simulink model "Urban_Air_Mobility_v3"  (R2021a)
settings: Solver=ode4  StartTime=0.0  StopTime=50  FixedStep=0.01  RelTol=1e-3
model workspace (MAT data in the model file):
  op_trim2 : handle (value not decoded)
undefined symbols (not defined in the file or in its folder): BackProp, Earth, ForwProp, geo, initialise, mass, simsetup, WGS84
libraries: dspindex x6, aerolibactuator x4, sharedutil x3, simulink x3, aerolibasang x2, aerolibtransform2 x2, aerolibutil x2, shared6dof x1, aerolibatmos2 x1, sharedtransform x1, aerolibconvert2 x1
(part 1 of 3)
settings Model: Creator=c109799  LastModifiedBy=gonza
settings SolverCC: AlgebraicLoopSolver=TrustRegion
settings DataIOCC: ExternalInput=getinputstruct(op_trim1)  InitialState=getstatestruct(op_trim1)  LoadExternalInput=on  LoadInitialState=on
settings DebuggingCC: SFMachineParentedDataDiag=warning  ArithmeticOperatorsInVariantConditions=warning
settings SFSimCC: CustomCodeUndefinedFunction=UseInterfaceOnly

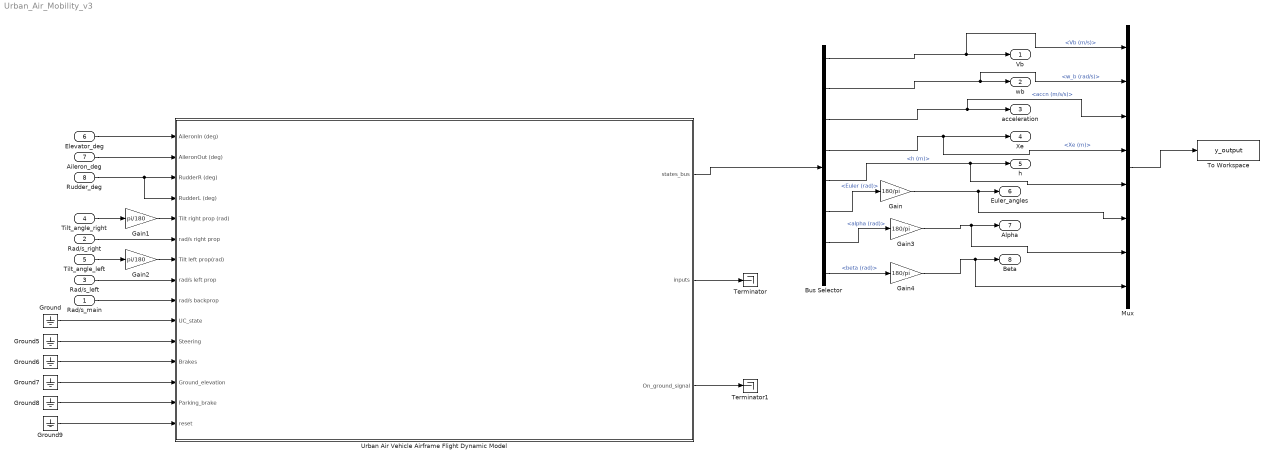
== system Urban_Air_Mobility_v3 ==
  Rad/s_main : Inport
  Rad/s_right : Inport  Port=2
  Rad/s_left : Inport  Port=3
  Tilt_angle_right : Inport  Port=4
  Tilt_angle_left : Inport  Port=5
  Elevator_deg : Inport  Port=6
  Aileron_deg : Inport  Port=7
  Rudder_deg : Inport  Port=8
  Bus Selector : BusSelector  OutputSignals=Vb (m/s),w_b (rad/s),accn (m/s/s),Xe (m),h (m),Euler (rad),alpha (rad),beta (rad)
  Gain : Gain  Gain=180/pi
  Gain1 : Gain  Gain=pi/180
  Gain2 : Gain  Gain=pi/180
  Gain3 : Gain  Gain=180/pi
  Gain4 : Gain  Gain=180/pi
  Ground{,5..9} (6 alike) : Ground
  Mux : Mux  Inputs=8
  Terminator : Terminator
  Terminator1 : Terminator
  To Workspace : ToWorkspace  VariableName=y_output  SampleTime=-1
  Urban Air Vehicle Airframe Flight Dynamic Model : Subsystem
  Vb : Outport  VectorParamsAs1DForOutWhenUnconnected=off
  wb : Outport  Port=2  VectorParamsAs1DForOutWhenUnconnected=off
  acceleration : Outport  Port=3  VectorParamsAs1DForOutWhenUnconnected=off
  Xe : Outport  Port=4  VectorParamsAs1DForOutWhenUnconnected=off
  h : Outport  Port=5  VectorParamsAs1DForOutWhenUnconnected=off
  Euler_angles : Outport  Port=6  VectorParamsAs1DForOutWhenUnconnected=off
  Alpha : Outport  Port=7  VectorParamsAs1DForOutWhenUnconnected=off
  Beta : Outport  Port=8  VectorParamsAs1DForOutWhenUnconnected=off
  wires:
  Ground/1 -> Urban Air Vehicle Airframe Flight Dynamic Model/10(UC_state)
  Ground5/1 -> Urban Air Vehicle Airframe Flight Dynamic Model/11(Steering)
  Ground6/1 -> Urban Air Vehicle Airframe Flight Dynamic Model/12(Brakes)
  Ground7/1 -> Urban Air Vehicle Airframe Flight Dynamic Model/13(Ground_elevation)
  Ground8/1 -> Urban Air Vehicle Airframe Flight Dynamic Model/14(Parking_brake)
  Ground9/1 -> Urban Air Vehicle Airframe Flight Dynamic Model/15("reset ")
  Urban Air Vehicle Airframe Flight Dynamic Model/1(states_bus) -> Bus Selector/1
  Urban Air Vehicle Airframe Flight Dynamic Model/2(inputs) -> Terminator/1
  Urban Air Vehicle Airframe Flight Dynamic Model/3(On_ground_signal) -> Terminator1/1
  Bus Selector/2 -> Mux/2, wb/1  "<w_b (rad/s)>"
  Bus Selector/5 -> Mux/5, h/1  "<h (m)>"
  Bus Selector/6 -> Gain/1  "<Euler (rad)>"
  Gain/1 -> Mux/6, Euler_angles/1
  Rudder_deg/1 -> Urban Air Vehicle Airframe Flight Dynamic Model/4("RudderL (deg) "), Urban Air Vehicle Airframe Flight Dynamic Model/3(RudderR (deg))
  Rad/s_main/1 -> Urban Air Vehicle Airframe Flight Dynamic Model/9(rad/s backprop)
  Rad/s_right/1 -> Urban Air Vehicle Airframe Flight Dynamic Model/6(rad/s right prop)
  Bus Selector/1 -> Mux/1, Vb/1  "<Vb (m/s)>"
  Bus Selector/3 -> Mux/3, acceleration/1  "<accn (m/s/s)>"
  Bus Selector/4 -> Mux/4, Xe/1  "<Xe (m)>"
  Aileron_deg/1 -> Urban Air Vehicle Airframe Flight Dynamic Model/2(AileronOut (deg))
  Elevator_deg/1 -> Urban Air Vehicle Airframe Flight Dynamic Model/1(AileronIn (deg))
  Gain1/1 -> Urban Air Vehicle Airframe Flight Dynamic Model/5(Tilt right prop (rad))
  Tilt_angle_right/1 -> Gain1/1
  Gain2/1 -> Urban Air Vehicle Airframe Flight Dynamic Model/7(Tilt left prop(rad))
  Tilt_angle_left/1 -> Gain2/1
  Bus Selector/7 -> Gain3/1  "<alpha (rad)>"
  Gain3/1 -> Mux/7, Alpha/1
  Bus Selector/8 -> Gain4/1  "<beta (rad)>"
  Gain4/1 -> Mux/8, Beta/1
  Mux/1 -> To Workspace/1
  Rad/s_left/1 -> Urban Air Vehicle Airframe Flight Dynamic Model/8(rad/s left prop)

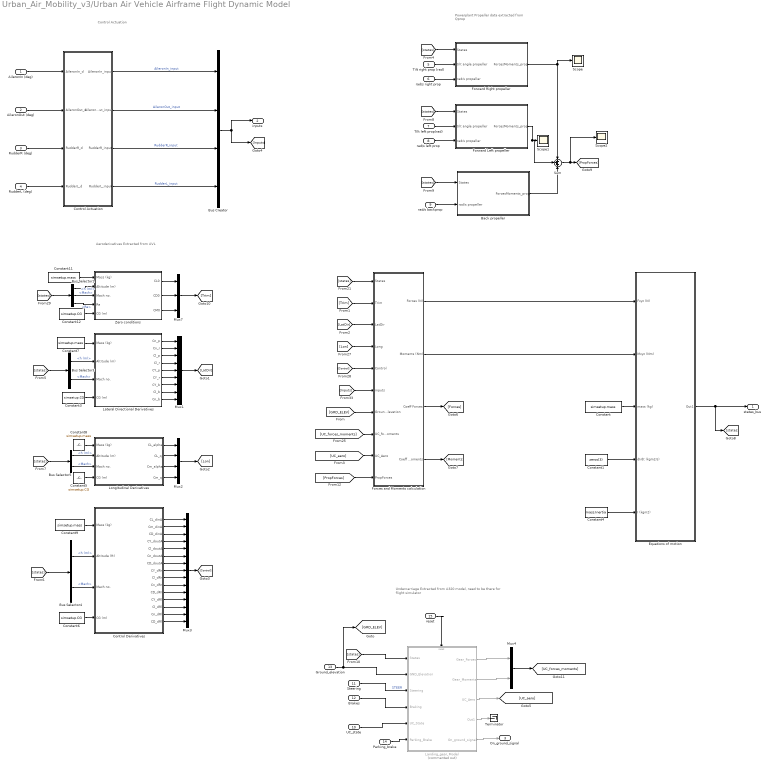
== system Urban_Air_Mobility_v3/Urban Air Vehicle Airframe Flight Dynamic Model ==
  note: Undercarriage
      | Extracted from A320 model, need to be there for flight simulator
  note: Control Actuation
  note: Aeroderivatives
      | Extracted from AVL
  note: Powerplant
      | Propeller data extracted from Qprop
  AileronIn (deg) : Inport
  AileronOut (deg) : Inport  Port=2
  RudderR (deg) : Inport  Port=3
  "RudderL (deg) " : Inport  Port=4
  Tilt right prop (rad) : Inport  Port=5
  rad/s right prop : Inport  Port=6
  Tilt left prop(rad) : Inport  Port=7
  rad/s left prop : Inport  Port=8
  rad/s backprop : Inport  Port=9
  UC_state : Inport  Port=10
  Steering : Inport  Port=11
  Brakes : Inport  Port=12
  Ground_elevation : Inport  Port=13
  Parking_brake : Inport  Port=14
  "reset " : Inport  Port=15
  Back propeller : Subsystem
  Bus Creator : BusCreator  Inputs=4
  Bus Selector1 : BusSelector  OutputSignals=h (m),Mach,Re
  Bus Selector3 : BusSelector  OutputSignals=h (m),Mach
  Bus Selector4 : BusSelector  OutputSignals=h (m),Mach
  Bus Selector5 : BusSelector  OutputSignals=h (m),Mach
  Constant{,7..9,11} (5 alike) : Constant  Value=simsetup.mass
  Constant1 : Constant  Value=zeros(3)
  Constant{3,5..6,12} (4 alike) : Constant  Value=simsetup.CG
  Constant4 : Constant  Value=mass.Inertia
  Control Actuation : Subsystem
  Control Derivatives : Subsystem
  Equations of motion : Subsystem
  Forces and Moments calculation : Subsystem
  Forward Left propeller : Subsystem
  Forward Right propeller : Subsystem
  Landing_gear_Model : Subsystem  Commented=on
  Lateral Directional Derivatives : Subsystem
  Longitudinal Derivatives : Subsystem
  Mux1 : Mux  Inputs=9
  Mux2 : Mux
  Mux3 : Mux  Inputs=15
  Mux4 : Mux  Inputs=2
  Mux7 : Mux  Inputs=3
  Scope : Scope
  Scope1 : Scope
  Scope2 : Scope
  Sum : Sum  Inputs=+++
  Terminator : Terminator
  Zero conditions : Subsystem
  states_bus : Outport  VectorParamsAs1DForOutWhenUnconnected=off
  inputs : Outport  Port=2  VectorParamsAs1DForOutWhenUnconnected=off
  On_ground_signal : Outport  Port=3  VectorParamsAs1DForOutWhenUnconnected=off
  wires:
  RudderR (deg)/1 -> Control Actuation/3(RudderR_d)
  Bus Creator/1 -> inputs/1, [Inputs]
  Lateral Directional Derivatives/5(CY_p) -> Mux1/5
  Lateral Directional Derivatives/6(CY_r) -> Mux1/6
  [states] -> Bus Selector4/1
  Bus Selector5/1 -> Longitudinal Derivatives/2(Altitude (m))  "<h (m)>"
  Mux2/1 -> [Lon]
  Bus Selector3/2 -> Lateral Directional Derivatives/3(Mach no.)  "<Mach>"
  Longitudinal Derivatives/4(Cm_q) -> Mux2/4
  Lateral Directional Derivatives/8(Cl_b) -> Mux1/8
  Bus Selector4/2 -> Control Derivatives/3(Mach no.)  "<Mach>"
  Lateral Directional Derivatives/4(Cl_r) -> Mux1/4
  Constant7/1 -> Lateral Directional Derivatives/1(Mass (kg))
  Lateral Directional Derivatives/3(Cl_p) -> Mux1/3
  Constant8/1 -> Longitudinal Derivatives/1(Mass (kg))
  Bus Selector3/1 -> Lateral Directional Derivatives/2(Altitude (m))  "<h (m)>"
  Bus Selector4/1 -> Control Derivatives/2(Altitude (ft))  "<h (m)>"
  [states] -> Bus Selector5/1
  Constant9/1 -> Control Derivatives/1(Mass (kg))
  Mux1/1 -> [LatDir]
  Longitudinal Derivatives/2(CL_q) -> Mux2/2
  Longitudinal Derivatives/3(Cm_alpha) -> Mux2/3
  Constant5/1 -> Longitudinal Derivatives/4(CG (m))
  Mux3/1 -> [Control]
  Lateral Directional Derivatives/1(Cn_p) -> Mux1/1
  Longitudinal Derivatives/1(CL_alpha) -> Mux2/1
  Lateral Directional Derivatives/7(CY_b) -> Mux1/7
  [states] -> Bus Selector3/1
  Constant6/1 -> Control Derivatives/4(CG (m))
  Constant3/1 -> Lateral Directional Derivatives/4(CG (m))
  Lateral Directional Derivatives/2(Cn_r) -> Mux1/2
  Bus Selector5/2 -> Longitudinal Derivatives/3(Mach no.)  "<Mach>"
  Equations of motion/1(Out1) -> [states], states_bus/1
  AileronIn (deg)/1 -> Control Actuation/1("AileronIn_d ")
  [UC_forces_moments] -> Forces and Moments calculation/8(UC_forces_moments)
  [Control] -> Forces and Moments calculation/5(Control)
  Forces and Moments calculation/4(Coeff Moments) -> [Moments]
  [Inputs] -> Forces and Moments calculation/6(inputs)
  [LatDir] -> Forces and Moments calculation/3(LatDir)
  Forces and Moments calculation/3(Coeff Forces) -> [Forces]
  [Lon] -> Forces and Moments calculation/4(Long)
  [Trim] -> Forces and Moments calculation/2(Trim)
  [states] -> Forces and Moments calculation/1(States)
  [states] -> Landing_gear_Model/1(States)
  Steering/1 -> Landing_gear_Model/3(Steering)  "STEER"
  Brakes/1 -> Landing_gear_Model/4(Braking)
  Ground_elevation/1 -> [GRD_ELEV], Landing_gear_Model/2(GND_Elevation)
  UC_state/1 -> Landing_gear_Model/5(UC_State)
  Mux4/1 -> [UC_forces_moments]
  Forces and Moments calculation/1(Forces (N)) -> Equations of motion/1(Fxyz (N))
  Forces and Moments calculation/2(Moments (Nm)) -> Equations of motion/2(Mxyz (Nm))
  Landing_gear_Model/3(UC_Aero) -> [UC_aero]
  Control Actuation/3(RudderR_input) -> Bus Creator/3  "RudderR_input"
  Landing_gear_Model/2(Gear_Moments) -> Mux4/2
  Landing_gear_Model/1(Gear_Forces) -> Mux4/1
  [GRD_ELEV] -> Forces and Moments calculation/7(Ground_Elevation)
  Parking_brake/1 -> Landing_gear_Model/6(Parking_Brake)
  Landing_gear_Model/5(On_ground_signal) -> On_ground_signal/1
  "reset "/1 -> Landing_gear_Model/Reset
  Landing_gear_Model/4(Out1) -> Terminator/1
  Constant/1 -> Equations of motion/3(mass (kg))
  Constant1/1 -> Equations of motion/4(dI/dt (kgm2/s))
  Constant4/1 -> Equations of motion/5(I (kgm2))
  [UC_aero] -> Forces and Moments calculation/9(UC_Aero)
  Lateral Directional Derivatives/9(Cn_b) -> Mux1/9
  Control Derivatives/1(CL_dinA) -> Mux3/1
  Control Derivatives/2(Cm_dinA) -> Mux3/2
  Control Derivatives/3(CD_dinA) -> Mux3/3
  AileronOut (deg)/1 -> Control Actuation/2(AileronOut_d)
  "RudderL (deg) "/1 -> Control Actuation/4("RudderL_d ")
  Control Actuation/1(AileronIn_input) -> Bus Creator/1  "AileronIn_input"
  Control Actuation/2(AileronOut_input) -> Bus Creator/2  "AileronOut_input"
  Control Actuation/4(RudderL_input) -> Bus Creator/4  "RudderL_input"
  Control Derivatives/4(CY_doutA) -> Mux3/4
  Control Derivatives/5(Cl_doutA) -> Mux3/5
  Control Derivatives/6(Cn_doutA) -> Mux3/6
  Control Derivatives/14(Cn_dRl) -> Mux3/14
  Control Derivatives/15(CD_dRl) -> Mux3/15
  Control Derivatives/13(Cl_dRl) -> Mux3/13
  Control Derivatives/12(CY_dRl) -> Mux3/12
  Control Derivatives/11(CD_dRr) -> Mux3/11
  Control Derivatives/10(Cn_dRr) -> Mux3/10
  Control Derivatives/9(Cl_dRr) -> Mux3/9
  Control Derivatives/8(CY_dRr) -> Mux3/8
  Control Derivatives/7(CD_doutA) -> Mux3/7
  [PropForces] -> Forces and Moments calculation/10(PropForces)
  Forward Right propeller/1(ForcesMoments_prop) -> Scope/1, Sum/1
  Forward Left propeller/1(ForcesMoments_prop) -> Sum/2, Scope1/1
  Sum/1 -> Scope2/1, [PropForces]
  [states] -> Forward Right propeller/1(States)
  Tilt left prop(rad)/1 -> Forward Left propeller/2(tilt angle propeller)
  rad/s right prop/1 -> Forward Right propeller/3(rad/s propeller)
  Tilt right prop (rad)/1 -> Forward Right propeller/2(tilt angle propeller)
  rad/s backprop/1 -> Back propeller/2(rad/s propeller)
  [states] -> Back propeller/1(States)
  rad/s left prop/1 -> Forward Left propeller/3(rad/s propeller)
  [states] -> Forward Left propeller/1(States)
  Back propeller/1(ForcesMoments_prop) -> Sum/3
  Zero conditions/3(CM0) -> Mux7/3
  Zero conditions/1(CL0) -> Mux7/1
  Bus Selector1/1 -> Zero conditions/2(Altitude (m))  "<h (m)>"
  Constant12/1 -> Zero conditions/5(CG (m))
  Zero conditions/2(CD0) -> Mux7/2
  [states] -> Bus Selector1/1
  Bus Selector1/2 -> Zero conditions/3(Mach no.)  "<Mach>"
  Mux7/1 -> [Trim]
  Bus Selector1/3 -> Zero conditions/4(Re)  "<Re>"
  Constant11/1 -> Zero conditions/1(Mass (kg))

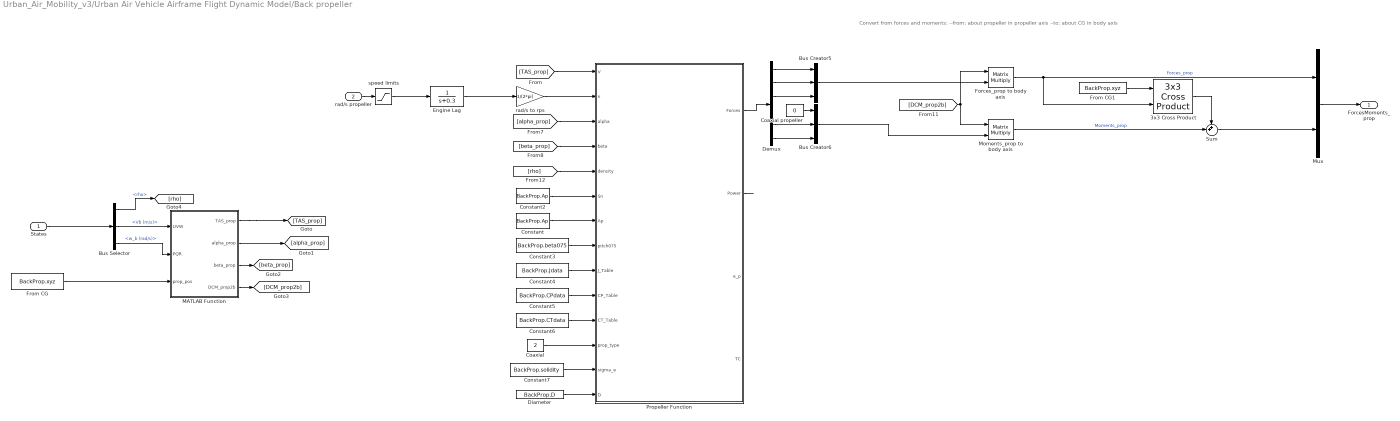
== system Urban_Air_Mobility_v3/Urban Air Vehicle Airframe Flight Dynamic Model/Back propeller ==
  note: Convert from forces and moments: --from: about propeller in propeller axis --to: about CG in body axis
  States : Inport
  rad/s propeller : Inport  Port=2
  3x3 Cross Product : sharedutil/3x3 Cross Product  aMode=aMode
      settings: SourceProductBaseCode=AE,PW,DR,MT,UV,VE
  Bus Creator5 : BusCreator  Inputs=3
  Bus Creator6 : BusCreator  Inputs=3
  Bus Selector : BusSelector  OutputSignals=rho,Vb (m/s),w_b (rad/s)
  "Coaxial " : Constant  Value=2
  Coaxial propeller : Constant  Value=0
  Constant : Constant  Value=BackProp.Ap
  Constant2 : Constant  Value=BackProp.Ap
  Constant3 : Constant  Value=BackProp.beta075
  Constant4 : Constant  Value=BackProp.Jdata
  Constant5 : Constant  Value=BackProp.CPdata
  Constant6 : Constant  Value=BackProp.CTdata
  Constant7 : Constant  Value=BackProp.solidity
  Demux : Demux  Outputs=6
  Diameter : Constant  Value=BackProp.D
  Engine Lag : TransferFcn  Denominator=[1 0.3]  ContinuousStateAttributes='EngineLag'
  Forces_prop to body axis : Product  Multiplication=Matrix(*)
  From CG : Constant  Value=BackProp.xyz
  From CG1 : Constant  Value=BackProp.xyz
  MATLAB Function : MATLAB Function  TreatAsAtomicUnit=on
  Moments_prop to body axis : Product  Multiplication=Matrix(*)
  Mux : Mux  Inputs=2
  Propeller Function : MATLAB Function  TreatAsAtomicUnit=on
  Sum : Sum  Inputs=++|
  rad/s to rps : Gain  Gain=1/(2*pi)
  speed limits : Saturate  UpperLimit=2000  LowerLimit=-1500
  ForcesMoments_prop : Outport
  wires:
  [rho] -> Propeller Function/5(density)
  MATLAB Function/2(alpha_prop) -> [alpha_prop]
  MATLAB Function/3(beta_prop) -> [beta_prop]
  MATLAB Function/1(TAS_prop) -> [TAS_prop]
  MATLAB Function/4(DCM_prop2b) -> [DCM_prop2b]
  [TAS_prop] -> Propeller Function/1(V)
  From CG/1 -> MATLAB Function/3(prop_pos)
  [alpha_prop] -> Propeller Function/3(alpha)
  rad/s propeller/1 -> speed limits/1
  States/1 -> Bus Selector/1
  Bus Selector/2 -> MATLAB Function/1(UVW)  "<Vb (m/s)>"
  Bus Selector/3 -> MATLAB Function/2(PQR)  "<w_b (rad/s)>"
  Bus Selector/1 -> [rho]  "<rho>"
  Mux/1 -> ForcesMoments_prop/1
  3x3 Cross Product/1 -> Sum/1
  Moments_prop to body axis/1 -> Sum/2  "Moments_prop"
  Forces_prop to body axis/1 -> 3x3 Cross Product/2, Mux/1  "Forces_prop"
  [DCM_prop2b] -> Forces_prop to body axis/1, Moments_prop to body axis/1
  From CG1/1 -> 3x3 Cross Product/1
  Bus Creator6/1 -> Moments_prop to body axis/2
  Sum/1 -> Mux/2
  [beta_prop] -> Propeller Function/4(beta)
  Constant/1 -> Propeller Function/7(Ap)
  Constant2/1 -> Propeller Function/6(Sn)
  Constant3/1 -> Propeller Function/8(pitch075)
  Constant4/1 -> Propeller Function/9(J_Table)
  Constant5/1 -> Propeller Function/10(CP_Table)
  Constant6/1 -> Propeller Function/11(CT_Table)
  Constant7/1 -> Propeller Function/13(sigma_e)
  "Coaxial "/1 -> Propeller Function/12(prop_type)
  Propeller Function/1(Forces) -> Demux/1
  Demux/1 -> Bus Creator5/1
  Demux/6 -> Bus Creator6/3
  Demux/2 -> Bus Creator5/2
  Demux/3 -> Bus Creator5/3
  Demux/5 -> Bus Creator6/2
  Propeller Function/2(Power) -> ?
  speed limits/1 -> Engine Lag/1
  Engine Lag/1 -> rad/s to rps/1
  Diameter/1 -> Propeller Function/14(D)
  rad/s to rps/1 -> Propeller Function/2(n)
  Coaxial propeller/1 -> Bus Creator6/1
  Bus Creator5/1 -> Forces_prop to body axis/2

== system Urban_Air_Mobility_v3/Urban Air Vehicle Airframe Flight Dynamic Model/Control Actuation ==
  "AileronIn_d " : Inport
  AileronOut_d : Inport  Port=2
  RudderR_d : Inport  Port=3
  "RudderL_d " : Inport  Port=4
  Aileron Actuator Transfer Function1 : aerolibactuator/Nonlinear Second-Order Actuator  wn_fin=45  z_fin=0.8  fin_max=25*pi/180  fin_min=-25*pi/180  fin_maxrate=100*pi/180  fin_act_0=0  fin_act_vel=0
      settings: SourceProductBaseCode=AE
  Aileron Actuator Transfer Function2 : aerolibactuator/Nonlinear Second-Order Actuator  wn_fin=45  z_fin=0.8  fin_max=25*pi/180  fin_min=-25*pi/180  fin_maxrate=100*pi/180  fin_act_0=0  fin_act_vel=0
      settings: SourceProductBaseCode=AE
  Rudder  Actuator Transfer Function1 : aerolibactuator/Nonlinear Second-Order Actuator  wn_fin=45  z_fin=0.8  fin_max=25*pi/180  fin_min=-25*pi/180  fin_maxrate=100*pi/180  fin_act_0=0  fin_act_vel=0
      settings: SourceProductBaseCode=AE
  Rudder  Actuator Transfer Function2 : aerolibactuator/Nonlinear Second-Order Actuator  wn_fin=45  z_fin=0.8  fin_max=25*pi/180  fin_min=-25*pi/180  fin_maxrate=100*pi/180  fin_act_0=0  fin_act_vel=0
      settings: SourceProductBaseCode=AE
  AileronIn_input : Outport  VectorParamsAs1DForOutWhenUnconnected=off
  AileronOut_input : Outport  Port=2  VectorParamsAs1DForOutWhenUnconnected=off
  RudderR_input : Outport  Port=3  VectorParamsAs1DForOutWhenUnconnected=off
  RudderL_input : Outport  Port=4  VectorParamsAs1DForOutWhenUnconnected=off
  wires:
  "AileronIn_d "/1 -> Aileron Actuator Transfer Function1/1
  RudderR_d/1 -> Rudder  Actuator Transfer Function1/1
  Aileron Actuator Transfer Function1/1 -> AileronIn_input/1  "Elevator_input"
  Rudder  Actuator Transfer Function1/1 -> RudderR_input/1
  AileronOut_d/1 -> Aileron Actuator Transfer Function2/1
  Aileron Actuator Transfer Function2/1 -> AileronOut_input/1  "Aileron_input"
  Rudder  Actuator Transfer Function2/1 -> RudderL_input/1
  "RudderL_d "/1 -> Rudder  Actuator Transfer Function2/1

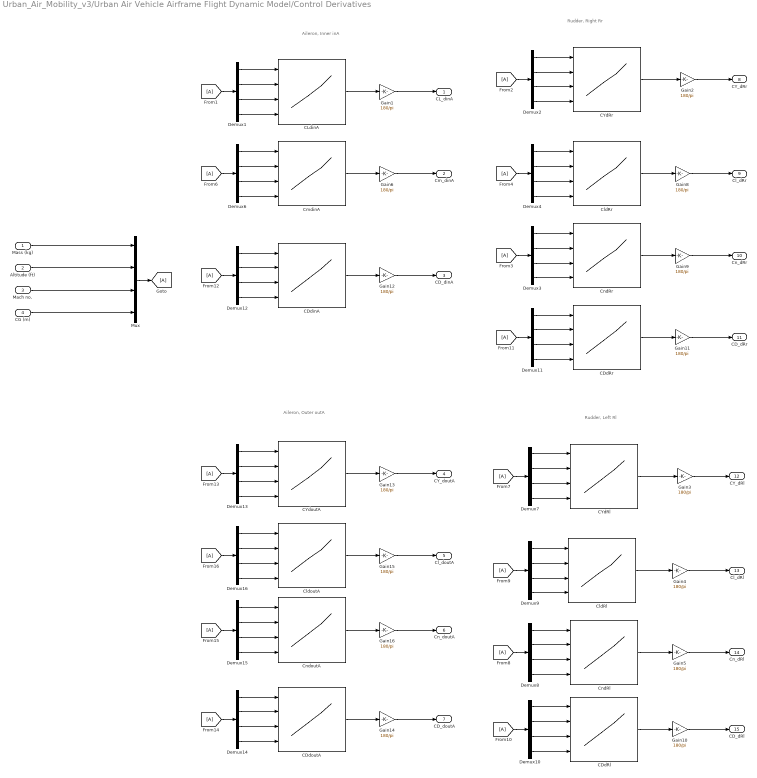
== system Urban_Air_Mobility_v3/Urban Air Vehicle Airframe Flight Dynamic Model/Control Derivatives ==
  note: Rudder, Right Rr
  note: Aileron, Inner inA
  note: Rudder, Left Rl
  note: Aileron, Outer outA
  Mass (kg) : Inport
  Altitude (ft) : Inport  Port=2
  Mach no. : Inport  Port=3
  CG (m) : Inport  Port=4
  CDdRl : Lookup_n-D  NumberOfTableDimensions=4  BreakpointsForDimension1=initialise.mass  BreakpointsForDimension2=initialise.Altitude  BreakpointsForDimension3=initialise.MLUT  BreakpointsForDimension4=initialise.CG  Table=initialise.CDdRl  InternalRulePriority=Speed  RndMeth=Simplest  InputSameDT=on
      settings: InputPortMap=u0,u1,u2,u3
  CDdRr : Lookup_n-D  NumberOfTableDimensions=4  BreakpointsForDimension1=initialise.mass  BreakpointsForDimension2=initialise.Altitude  BreakpointsForDimension3=initialise.MLUT  BreakpointsForDimension4=initialise.CG  Table=initialise.CDdRr  InternalRulePriority=Speed  RndMeth=Simplest  InputSameDT=on
      settings: InputPortMap=u0,u1,u2,u3
  CDdinA : Lookup_n-D  NumberOfTableDimensions=4  BreakpointsForDimension1=initialise.mass  BreakpointsForDimension2=initialise.Altitude  BreakpointsForDimension3=initialise.MLUT  BreakpointsForDimension4=initialise.CG  Table=initialise.CDdinA  InternalRulePriority=Speed  RndMeth=Simplest  InputSameDT=on
      settings: InputPortMap=u0,u1,u2,u3
  CDdoutA : Lookup_n-D  NumberOfTableDimensions=4  BreakpointsForDimension1=initialise.mass  BreakpointsForDimension2=initialise.Altitude  BreakpointsForDimension3=initialise.MLUT  BreakpointsForDimension4=initialise.CG  Table=initialise.CDdoutA  InternalRulePriority=Speed  RndMeth=Simplest  InputSameDT=on
      settings: InputPortMap=u0,u1,u2,u3
  CLdinA : Lookup_n-D  NumberOfTableDimensions=4  BreakpointsForDimension1=initialise.mass  BreakpointsForDimension2=initialise.Altitude  BreakpointsForDimension3=initialise.MLUT  BreakpointsForDimension4=initialise.CG  Table=initialise.CLdinA  InternalRulePriority=Speed  RndMeth=Simplest  InputSameDT=on
      settings: InputPortMap=u0,u1,u2,u3
  CYdRl : Lookup_n-D  NumberOfTableDimensions=4  BreakpointsForDimension1=initialise.mass  BreakpointsForDimension2=initialise.Altitude  BreakpointsForDimension3=initialise.MLUT  BreakpointsForDimension4=initialise.CG  Table=initialise.CYdRl  InternalRulePriority=Speed  RndMeth=Simplest  InputSameDT=on
      settings: InputPortMap=u0,u1,u2,u3
  CYdRr : Lookup_n-D  NumberOfTableDimensions=4  BreakpointsForDimension1=initialise.mass  BreakpointsForDimension2=initialise.Altitude  BreakpointsForDimension3=initialise.MLUT  BreakpointsForDimension4=initialise.CG  Table=initialise.CYdRr  InternalRulePriority=Speed  RndMeth=Simplest  InputSameDT=on
      settings: InputPortMap=u0,u1,u2,u3
  CYdoutA : Lookup_n-D  NumberOfTableDimensions=4  BreakpointsForDimension1=initialise.mass  BreakpointsForDimension2=initialise.Altitude  BreakpointsForDimension3=initialise.MLUT  BreakpointsForDimension4=initialise.CG  Table=initialise.CYdoutA  InternalRulePriority=Speed  RndMeth=Simplest  InputSameDT=on
      settings: InputPortMap=u0,u1,u2,u3
  CldRl : Lookup_n-D  NumberOfTableDimensions=4  BreakpointsForDimension1=initialise.mass  BreakpointsForDimension2=initialise.Altitude  BreakpointsForDimension3=initialise.MLUT  BreakpointsForDimension4=initialise.CG  Table=initialise.CldRl  InternalRulePriority=Speed  RndMeth=Simplest  InputSameDT=on
      settings: InputPortMap=u0,u1,u2,u3
  CldRr : Lookup_n-D  NumberOfTableDimensions=4  BreakpointsForDimension1=initialise.mass  BreakpointsForDimension2=initialise.Altitude  BreakpointsForDimension3=initialise.MLUT  BreakpointsForDimension4=initialise.CG  Table=initialise.CldRr  InternalRulePriority=Speed  RndMeth=Simplest  InputSameDT=on
      settings: InputPortMap=u0,u1,u2,u3
  CldoutA : Lookup_n-D  NumberOfTableDimensions=4  BreakpointsForDimension1=initialise.mass  BreakpointsForDimension2=initialise.Altitude  BreakpointsForDimension3=initialise.MLUT  BreakpointsForDimension4=initialise.CG  Table=initialise.CldoutA  InternalRulePriority=Speed  RndMeth=Simplest  InputSameDT=on
      settings: InputPortMap=u0,u1,u2,u3
  CmdinA : Lookup_n-D  NumberOfTableDimensions=4  BreakpointsForDimension1=initialise.mass  BreakpointsForDimension2=initialise.Altitude  BreakpointsForDimension3=initialise.MLUT  BreakpointsForDimension4=initialise.CG  Table=initialise.CmdinA  InternalRulePriority=Speed  RndMeth=Simplest  InputSameDT=on
      settings: InputPortMap=u0,u1,u2,u3
  CndRl : Lookup_n-D  NumberOfTableDimensions=4  BreakpointsForDimension1=initialise.mass  BreakpointsForDimension2=initialise.Altitude  BreakpointsForDimension3=initialise.MLUT  BreakpointsForDimension4=initialise.CG  Table=initialise.CndRl  InternalRulePriority=Speed  RndMeth=Simplest  InputSameDT=on
      settings: InputPortMap=u0,u1,u2,u3
  CndRr : Lookup_n-D  NumberOfTableDimensions=4  BreakpointsForDimension1=initialise.mass  BreakpointsForDimension2=initialise.Altitude  BreakpointsForDimension3=initialise.MLUT  BreakpointsForDimension4=initialise.CG  Table=initialise.CndRr  InternalRulePriority=Speed  RndMeth=Simplest  InputSameDT=on
      settings: InputPortMap=u0,u1,u2,u3
  CndoutA : Lookup_n-D  NumberOfTableDimensions=4  BreakpointsForDimension1=initialise.mass  BreakpointsForDimension2=initialise.Altitude  BreakpointsForDimension3=initialise.MLUT  BreakpointsForDimension4=initialise.CG  Table=initialise.CndoutA  InternalRulePriority=Speed  RndMeth=Simplest  InputSameDT=on
      settings: InputPortMap=u0,u1,u2,u3
  Demux{1..4,6..16} (15 alike) : Demux
  Gain{1..6,8..16} (15 alike) : Gain  Gain=180/pi
  Mux : Mux
  CL_dinA : Outport  VectorParamsAs1DForOutWhenUnconnected=off
  Cm_dinA : Outport  Port=2  VectorParamsAs1DForOutWhenUnconnected=off
  CD_dinA : Outport  Port=3  VectorParamsAs1DForOutWhenUnconnected=off
  CY_doutA : Outport  Port=4  VectorParamsAs1DForOutWhenUnconnected=off
  Cl_doutA : Outport  Port=5  VectorParamsAs1DForOutWhenUnconnected=off
  Cn_doutA : Outport  Port=6  VectorParamsAs1DForOutWhenUnconnected=off
  CD_doutA : Outport  Port=7  VectorParamsAs1DForOutWhenUnconnected=off
  CY_dRr : Outport  Port=8  VectorParamsAs1DForOutWhenUnconnected=off
  Cl_dRr : Outport  Port=9  VectorParamsAs1DForOutWhenUnconnected=off
  Cn_dRr : Outport  Port=10  VectorParamsAs1DForOutWhenUnconnected=off
  CD_dRr : Outport  Port=11  VectorParamsAs1DForOutWhenUnconnected=off
  CY_dRl : Outport  Port=12  VectorParamsAs1DForOutWhenUnconnected=off
  Cl_dRl : Outport  Port=13  VectorParamsAs1DForOutWhenUnconnected=off
  Cn_dRl : Outport  Port=14  VectorParamsAs1DForOutWhenUnconnected=off
  CD_dRl : Outport  Port=15  VectorParamsAs1DForOutWhenUnconnected=off
  wires:
  Mass (kg)/1 -> Mux/1
  Mach no./1 -> Mux/3
  CG (m)/1 -> Mux/4
  Mux/1 -> [A]
  Demux3/1 -> CndRr/1
  Demux3/3 -> CndRr/3
  Demux3/4 -> CndRr/4
  Demux3/2 -> CndRr/2
  [A] -> Demux3/1
  Demux4/1 -> CldRr/1
  Demux4/3 -> CldRr/3
  Demux4/4 -> CldRr/4
  Demux4/2 -> CldRr/2
  [A] -> Demux4/1
  CldRr/1 -> Gain8/1
  CndRr/1 -> Gain9/1
  Gain8/1 -> Cl_dRr/1
  Gain9/1 -> Cn_dRr/1
  Altitude (ft)/1 -> Mux/2
  Demux6/4 -> CmdinA/4
  Gain6/1 -> Cm_dinA/1
  [A] -> Demux6/1
  Demux6/3 -> CmdinA/3
  Demux6/1 -> CmdinA/1
  CmdinA/1 -> Gain6/1
  Demux6/2 -> CmdinA/2
  Demux1/3 -> CLdinA/3
  Demux1/4 -> CLdinA/4
  Demux1/1 -> CLdinA/1
  [A] -> Demux1/1
  CLdinA/1 -> Gain1/1
  Demux1/2 -> CLdinA/2
  Gain1/1 -> CL_dinA/1
  Demux2/2 -> CYdRr/2
  Gain2/1 -> CY_dRr/1
  Demux2/4 -> CYdRr/4
  [A] -> Demux2/1
  CYdRr/1 -> Gain2/1
  Demux2/3 -> CYdRr/3
  Demux2/1 -> CYdRr/1
  CndRl/1 -> Gain5/1
  Demux9/1 -> CldRl/1
  Gain5/1 -> Cn_dRl/1
  Demux8/4 -> CndRl/4
  [A] -> Demux8/1
  Gain4/1 -> Cl_dRl/1
  CldRl/1 -> Gain4/1
  Demux8/2 -> CndRl/2
  Demux9/4 -> CldRl/4
  [A] -> Demux9/1
  Demux8/3 -> CndRl/3
  Demux8/1 -> CndRl/1
  Demux9/2 -> CldRl/2
  Demux9/3 -> CldRl/3
  Demux7/2 -> CYdRl/2
  [A] -> Demux7/1
  CYdRl/1 -> Gain3/1
  Demux7/1 -> CYdRl/1
  Demux7/4 -> CYdRl/4
  Gain3/1 -> CY_dRl/1
  Demux7/3 -> CYdRl/3
  Demux10/1 -> CDdRl/1
  CDdRl/1 -> Gain10/1
  [A] -> Demux10/1
  Demux10/2 -> CDdRl/2
  Gain10/1 -> CD_dRl/1
  Demux10/4 -> CDdRl/4
  Demux10/3 -> CDdRl/3
  Gain11/1 -> CD_dRr/1
  Demux11/4 -> CDdRr/4
  CDdRr/1 -> Gain11/1
  Demux11/1 -> CDdRr/1
  [A] -> Demux11/1
  Demux11/3 -> CDdRr/3
  Demux11/2 -> CDdRr/2
  Demux12/2 -> CDdinA/2
  CDdinA/1 -> Gain12/1
  Demux12/4 -> CDdinA/4
  Demux12/3 -> CDdinA/3
  Gain12/1 -> CD_dinA/1
  Demux12/1 -> CDdinA/1
  [A] -> Demux12/1
  CDdoutA/1 -> Gain14/1
  [A] -> Demux14/1
  CYdoutA/1 -> Gain13/1
  Demux15/3 -> CndoutA/3
  Gain14/1 -> CD_doutA/1
  Demux14/2 -> CDdoutA/2
  Demux16/4 -> CldoutA/4
  Demux14/3 -> CDdoutA/3
  Demux15/2 -> CndoutA/2
  Demux16/2 -> CldoutA/2
  Demux16/3 -> CldoutA/3
  Demux13/1 -> CYdoutA/1
  Demux13/2 -> CYdoutA/2
  Demux16/1 -> CldoutA/1
  Gain13/1 -> CY_doutA/1
  [A] -> Demux15/1
  CldoutA/1 -> Gain15/1
  Demux13/3 -> CYdoutA/3
  CndoutA/1 -> Gain16/1
  [A] -> Demux13/1
  Gain16/1 -> Cn_doutA/1
  Demux14/1 -> CDdoutA/1
  Demux13/4 -> CYdoutA/4
  Demux14/4 -> CDdoutA/4
  Demux15/1 -> CndoutA/1
  Demux15/4 -> CndoutA/4
  [A] -> Demux16/1
  Gain15/1 -> Cl_doutA/1

== system Urban_Air_Mobility_v3/Urban Air Vehicle Airframe Flight Dynamic Model/Equations of motion ==
  Fxyz (N) : Inport
  Mxyz (Nm) : Inport  Port=2
  mass (kg) : Inport  Port=3
  dI/dt (kgm2/s) : Inport  Port=4
  I (kgm2) : Inport  Port=5
  Bus Creator : BusCreator  Inputs=18
  Constant : Constant  Value=0
  Custom Variable Mass 6DOF (Euler Angles) : shared6dof/6DOF (Euler Angles)  units=Metric (MKS)  mtype=Custom Variable  rep=Euler Angles  xme_0=simsetup.initialXYZ  Vm_0=simsetup.initialUVW  eul_0=simsetup.initialEuler  pm_0=[0 0 0]  mass_0=1.0  mass_e=0.5  mass_f=2.0  inertia=eye(3)  inertia_e=eye(3)  inertia_f=2*eye(3)  k_quat=1.0  vre_flag=off  abi_flag=off  aMode=0  xme_statename={'Xe', 'Ye', 'Ze'}  Vm_statename={'U', 'v', 'w'}  eul_statename={'phi', 'theta', 'psi'}  quat_statename=''  pm_statename={'p', 'q', 'r'}  mass_statename=''
      settings: SourceProductBaseCode=AE,PW,DR,MT,UV,VE
  Divide : Product  Inputs=**/
  Dynamic Pressure : aerolibasang/Dynamic Pressure
  Dynamic Viscosity : Lookup_n-D  NumberOfTableDimensions=1  BreakpointsForDimension1=initialise.alt  BreakpointsForDimension2=initialise.Altitude  BreakpointsForDimension3=initialise.MLUT  BreakpointsForDimension4=initialise.CG  Table=initialise.dyn_visc  InternalRulePriority=Speed  RndMeth=Simplest  InputSameDT=on
  Flat Earth to LLA1 : aerolibtransform2/Flat Earth to LLA  units=Metric (MKS)  ptype=Earth (WGS84)  F=1/298.257223563  R=6378137  refPosPort=off  LL0=simsetup.initialLatLong  psi=0
  Gain : Gain  Gain=-1
  ISA Atmosphere Model : aerolibatmos2/ISA Atmosphere Model  custom=off  g=9.80665  gamma=1.4  R=287.0531  L=0.0065  h_trop=11000  h_strat=20000  rho0=1.225  P0=101325  T0=288.15  h0=0
  "Incidence, Sideslip, & Airspeed2" : MATLAB Function  TreatAsAtomicUnit=on
  Mach Number : aerolibasang/Mach Number
      settings: SourceProductBaseCode=AE
  Scope : Scope
  Scope1 : Scope
  Scope2 : Scope
  Selector : Selector  InputPortWidth=3  IndexOptions=Index vector (dialog)  Indices=3  OutputSizes=1
  Terminator1 : Terminator
  Terminator2 : Terminator
  Out1 : Outport  VectorParamsAs1DForOutWhenUnconnected=off
  wires:
  Custom Variable Mass 6DOF (Euler Angles)/6 -> Bus Creator/6  "w_b (rad/s)"
  ISA Atmosphere Model/2 -> Mach Number/2
  Custom Variable Mass 6DOF (Euler Angles)/5 -> Bus Creator/5, Dynamic Pressure/1, Mach Number/1, "Incidence, Sideslip, & Airspeed2"/1(V_body)  "Vb (m/s)"
  Selector/1 -> Gain/1
  Dynamic Pressure/1 -> Bus Creator/14  "q_dyn (Pa)"
  ISA Atmosphere Model/3 -> Terminator2/1
  Bus Creator/1 -> Out1/1
  Mxyz (Nm)/1 -> Custom Variable Mass 6DOF (Euler Angles)/2
  ISA Atmosphere Model/4 -> Bus Creator/18, Divide/2, Dynamic Pressure/2  "rho"
  I (kgm2)/1 -> Custom Variable Mass 6DOF (Euler Angles)/5
  mass (kg)/1 -> Custom Variable Mass 6DOF (Euler Angles)/3
  Flat Earth to LLA1/1 -> Bus Creator/16  "Lat_Long"
  ISA Atmosphere Model/1 -> Bus Creator/12  "Tamb"
  Constant/1 -> Flat Earth to LLA1/2
  Custom Variable Mass 6DOF (Euler Angles)/8 -> Bus Creator/8  "accn (m/s/s)"
  Gain/1 -> Dynamic Viscosity/1, Bus Creator/15, ISA Atmosphere Model/1  "h (m)"
  "Incidence, Sideslip, & Airspeed2"/2(beta) -> Bus Creator/10  "beta (rad)"
  Custom Variable Mass 6DOF (Euler Angles)/3 -> Scope1/1, Bus Creator/3  "Euler (rad)"
  Custom Variable Mass 6DOF (Euler Angles)/7 -> Bus Creator/7  "w_b_dot (rad/s/s)"
  Mach Number/1 -> Bus Creator/13  "Mach"
  Custom Variable Mass 6DOF (Euler Angles)/1 -> Scope2/1, Bus Creator/1  "Ve (m/s)"
  Custom Variable Mass 6DOF (Euler Angles)/4 -> Bus Creator/4  "DCMbe"
  Custom Variable Mass 6DOF (Euler Angles)/2 -> Scope/1, Bus Creator/2, Flat Earth to LLA1/1, Selector/1  "Xe (m)"
  "Incidence, Sideslip, & Airspeed2"/3(VTAS) -> Divide/1, Bus Creator/11  "VTAS (m/s)"
  "Incidence, Sideslip, & Airspeed2"/1(alpha) -> Bus Creator/9  "alpha (rad)"
  Flat Earth to LLA1/2 -> Terminator1/1
  dI/dt (kgm2/s)/1 -> Custom Variable Mass 6DOF (Euler Angles)/4
  Dynamic Viscosity/1 -> Divide/3  "dyn_visc"
  Divide/1 -> Bus Creator/17  "Re"
  Fxyz (N)/1 -> Custom Variable Mass 6DOF (Euler Angles)/1

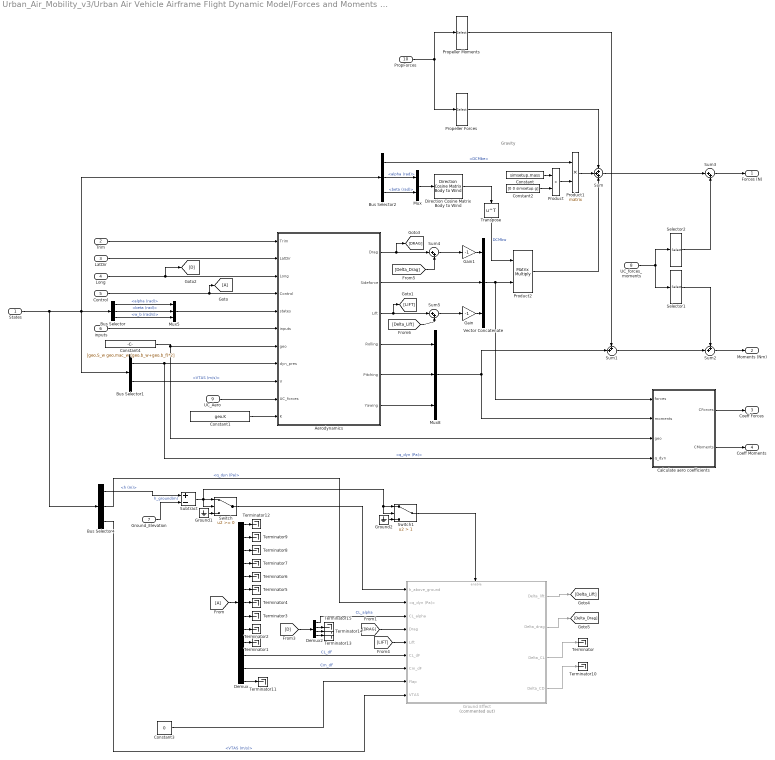
== system Urban_Air_Mobility_v3/Urban Air Vehicle Airframe Flight Dynamic Model/Forces and Moments calculation ==
  note: Gravity
  States : Inport
  Trim : Inport  Port=2
  LatDir : Inport  Port=3
  Long : Inport  Port=4
  Control : Inport  Port=5
  inputs : Inport  Port=6
  Ground_Elevation : Inport  Port=7
  UC_forces_moments : Inport  Port=8
  UC_Aero : Inport  Port=9
  PropForces : Inport  Port=10
  Aerodynamics : MATLAB Function  TreatAsAtomicUnit=on
  Bus Selector : BusSelector  OutputSignals=alpha (rad),beta (rad),w_b (rad/s)
  Bus Selector1 : BusSelector  OutputSignals=q_dyn (Pa),VTAS (m/s)
  Bus Selector2 : BusSelector  OutputSignals=DCMbe,alpha (rad),beta (rad)
  Bus Selector4 : BusSelector  OutputSignals=h (m),q_dyn (Pa),VTAS (m/s)
  Calculate aero coefficients : MATLAB Function  TreatAsAtomicUnit=on
  Constant : Constant  Value=simsetup.mass
  Constant1 : Constant  Value=geo.K
  Constant2 : Constant  Value=[0 0 simsetup.g]
  Constant3 : Constant  Value=0
  Constant4 : Constant  Value=[geo.S_w geo.mac_w (geo.b_w+geo.b_f)*2]
  Demux : Demux  Outputs=13
  Demux2 : Demux
  Direction Cosine Matrix Body to Wind : aerolibtransform2/Direction Cosine Matrix Body to Wind
      settings: SourceProductBaseCode=AE
  Gain : Gain  Gain=-1
  Gain1 : Gain  Gain=-1
  "Ground Effect " : Subsystem  Commented=on
  Ground1 : Ground
  Ground2 : Ground
  Mux : Mux  Inputs=2
  Mux5 : Mux  Inputs=3
  Mux8 : Mux  Inputs=3
  Product : Product
  Product1 : Product  Multiplication=Matrix(*)
  Product2 : Product  Multiplication=Matrix(*)
  Propeller Forces : Selector  InputPortWidth=6  IndexOptions=Index vector (dialog)  Indices=[1 2 3]  OutputSizes=1
  Propeller Moments : Selector  InputPortWidth=6  IndexOptions=Index vector (dialog)  Indices=[4 5 6]  OutputSizes=1
  Selector1 : Selector  InputPortWidth=6  IndexOptions=Index vector (dialog)  Indices=[4 5 6]  OutputSizes=1
  Selector2 : Selector  InputPortWidth=6  IndexOptions=Index vector (dialog)  Indices=[1 2 3]  OutputSizes=1
  Subtract : Sum  Inputs=+-
  Sum : Sum  Inputs=+++
  Sum1 : Sum  Inputs=++|
  Sum2 : Sum  Inputs=++|
  Sum3 : Sum  Inputs=|++
  Sum4 : Sum  Inputs=|++
  Sum5 : Sum  Inputs=|++
  Switch : Switch
  Switch1 : Switch  Criteria=u2 > Threshold  Threshold=1
  Terminator{,1..15} (16 alike) : Terminator
  Transpose : Math  Operator=transpose  SignedPower=on  SaturateOnIntegerOverflow=on
  Vector Concatenate : Concatenate  NumInputs=3
  Forces (N) : Outport  VectorParamsAs1DForOutWhenUnconnected=off
  Moments (Nm) : Outport  Port=2  VectorParamsAs1DForOutWhenUnconnected=off
  Coeff Forces : Outport  Port=3  VectorParamsAs1DForOutWhenUnconnected=off
  Coeff Moments : Outport  Port=4  VectorParamsAs1DForOutWhenUnconnected=off
  wires:
  LatDir/1 -> Aerodynamics/2(LatDir)
  Long/1 -> Aerodynamics/3(Long), [D]
  Control/1 -> Aerodynamics/4(Control), [A]
  Trim/1 -> Aerodynamics/1(Trim)
  Bus Selector/3 -> Mux5/3  "<w_b (rad/s)>"
  Bus Selector/2 -> Mux5/2  "<beta (rad)>"
  Bus Selector/1 -> Mux5/1  "<alpha (rad)>"
  inputs/1 -> Aerodynamics/6(inputs)
  Aerodynamics/6(Yawing) -> Mux8/3
  Aerodynamics/4(Rolling) -> Mux8/1
  Mux5/1 -> Aerodynamics/5(states)
  Constant4/1 -> Aerodynamics/7(geo), Calculate aero coefficients/3(geo)
  Bus Selector1/1 -> Aerodynamics/8(dyn_pres), Calculate aero coefficients/4(q_dyn)  "<q_dyn (Pa)>"
  Bus Selector1/2 -> Aerodynamics/9(V)  "<VTAS (m/s)>"
  Calculate aero coefficients/2(CMoments) -> Coeff Moments/1
  Calculate aero coefficients/1(CForces) -> Coeff Forces/1
  Vector Concatenate/1 -> Calculate aero coefficients/1(forces), Product2/2
  Constant2/1 -> Product/2
  Aerodynamics/1(Drag) -> Sum4/1, [DRAG]
  Product2/1 -> Sum/3
  Bus Selector2/1 -> Product1/1  "<DCMbe>"
  Bus Selector2/3 -> Mux/2  "<beta (rad)>"
  Gain/1 -> Vector Concatenate/3
  Aerodynamics/3(Lift) -> Sum5/1, [LIFT]
  Product1/1 -> Sum/2
  Aerodynamics/2(Sideforce) -> Vector Concatenate/2
  Bus Selector2/2 -> Mux/1  "<alpha (rad)>"
  Gain1/1 -> Vector Concatenate/1
  Constant/1 -> Product/1
  States/1 -> Bus Selector2/1, Bus Selector1/1, Bus Selector/1, Bus Selector4/1
  Mux/1 -> Direction Cosine Matrix Body to Wind/1
  Product/1 -> Product1/2
  Mux8/1 -> Calculate aero coefficients/2(moments), Sum1/2
  Aerodynamics/5(Pitching) -> Mux8/2
  Direction Cosine Matrix Body to Wind/1 -> Transpose/1
  Transpose/1 -> Product2/1  "DCMbw"
  UC_Aero/1 -> Aerodynamics/10(UC_forces)
  Sum2/1 -> Moments (Nm)/1
  Sum3/1 -> Forces (N)/1
  Selector2/1 -> Sum3/2
  Selector1/1 -> Sum2/1
  Sum1/1 -> Sum2/2
  Sum/1 -> Sum3/1
  UC_forces_moments/1 -> Selector1/1, Selector2/1
  Demux/13 -> Terminator11/1
  [A] -> Demux/1
  Demux/10 -> Terminator1/1
  Demux/9 -> Terminator2/1
  Demux/8 -> Terminator3/1
  Demux/7 -> Terminator4/1
  Demux/6 -> Terminator5/1
  Demux/5 -> Terminator6/1
  Demux/4 -> Terminator7/1
  Demux/3 -> Terminator8/1
  Demux/2 -> Terminator9/1
  Demux/1 -> Terminator12/1
  Ground_Elevation/1 -> Subtract/2  "h_ground(m)"
  Bus Selector4/1 -> Subtract/1  "<h (m)>"
  [D] -> Demux2/1
  Demux2/4 -> Terminator13/1
  Demux2/3 -> Terminator14/1
  Demux2/2 -> Terminator15/1
  Sum4/1 -> Gain1/1
  [Delta_Drag] -> Sum4/2
  Sum5/1 -> Gain/1
  [Delta_Lift] -> Sum5/2
  Subtract/1 -> Switch1/2, Switch1/1, Switch/2, Switch/1
  Ground1/1 -> Switch/3
  Switch/1 -> "Ground Effect "/1(h_above_ground)
  Bus Selector4/2 -> "Ground Effect "/2(<q_dyn (Pa)>)  "<q_dyn (Pa)>"
  Demux2/1 -> "Ground Effect "/3(CL_alpha)  "CL_alpha"
  [DRAG] -> "Ground Effect "/4(Drag)
  [LIFT] -> "Ground Effect "/5(Lift)
  Demux/11 -> "Ground Effect "/6(CL_dF)  "CL_dF"
  Demux/12 -> "Ground Effect "/7(Cm_dF)  "Cm_dF"
  "Ground Effect "/1("Delta_lift ") -> [Delta_Lift]
  "Ground Effect "/2(Delta_drag) -> [Delta_Drag]
  Switch1/1 -> "Ground Effect "/Enable
  Ground2/1 -> Switch1/3
  "Ground Effect "/3(Delta_CL) -> Terminator/1
  "Ground Effect "/4("Delta_CD ") -> Terminator10/1
  Constant3/1 -> "Ground Effect "/8(Flap)
  Bus Selector4/3 -> "Ground Effect "/9(VTAS)  "<VTAS (m/s)>"
  PropForces/1 -> Propeller Moments/1, Propeller Forces/1
  Propeller Forces/1 -> Sum/1
  Propeller Moments/1 -> Sum1/1
  Constant1/1 -> Aerodynamics/11(K)

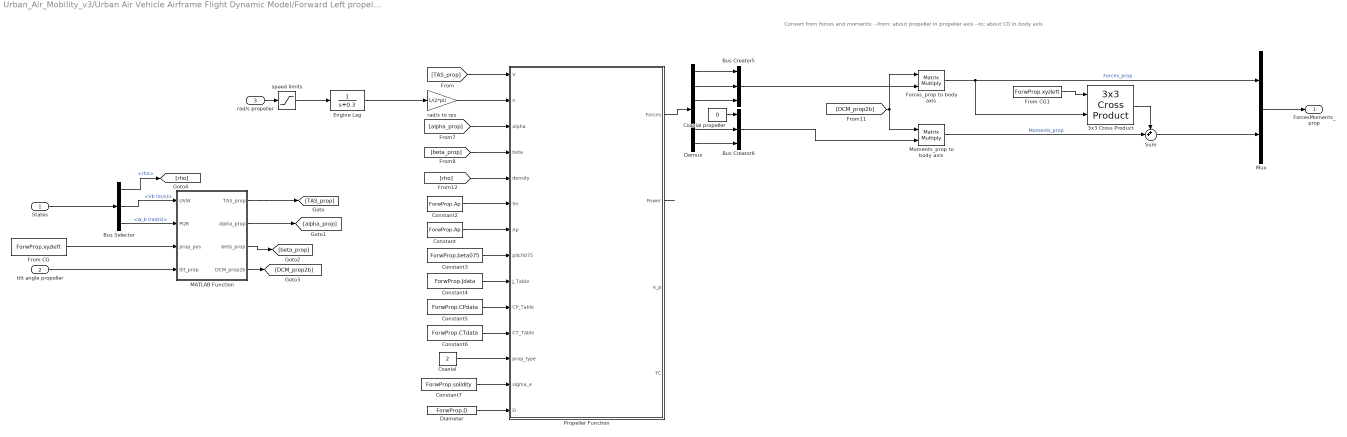
== system Urban_Air_Mobility_v3/Urban Air Vehicle Airframe Flight Dynamic Model/Forward Left propeller ==
  note: Convert from forces and moments: --from: about propeller in propeller axis --to: about CG in body axis
  States : Inport
  tilt angle propeller : Inport  Port=2
  rad/s propeller : Inport  Port=3
  3x3 Cross Product : sharedutil/3x3 Cross Product  aMode=aMode
      settings: SourceProductBaseCode=AE,PW,DR,MT,UV,VE
  Bus Creator5 : BusCreator  Inputs=3
  Bus Creator6 : BusCreator  Inputs=3
  Bus Selector : BusSelector  OutputSignals=rho,Vb (m/s),w_b (rad/s)
  "Coaxial " : Constant  Value=2
  Coaxial propeller : Constant  Value=0
  Constant : Constant  Value=ForwProp.Ap
  Constant2 : Constant  Value=ForwProp.Ap
  Constant3 : Constant  Value=ForwProp.beta075
  Constant4 : Constant  Value=ForwProp.Jdata
  Constant5 : Constant  Value=ForwProp.CPdata
  Constant6 : Constant  Value=ForwProp.CTdata
  Constant7 : Constant  Value=ForwProp.solidity
  Demux : Demux  Outputs=6
  Diameter : Constant  Value=ForwProp.D
  Engine Lag : TransferFcn  Denominator=[1 0.3]  ContinuousStateAttributes='EngineLag'
  Forces_prop to body axis : Product  Multiplication=Matrix(*)
  From CG : Constant  Value=ForwProp.xyzleft
  From CG1 : Constant  Value=ForwProp.xyzleft
  MATLAB Function : MATLAB Function  TreatAsAtomicUnit=on
  Moments_prop to body axis : Product  Multiplication=Matrix(*)
  Mux : Mux  Inputs=2
  Propeller Function : MATLAB Function  TreatAsAtomicUnit=on
  Sum : Sum  Inputs=++|
  rad/s to rps : Gain  Gain=1/(2*pi)
  speed limits : Saturate  UpperLimit=2000  LowerLimit=-1500
  ForcesMoments_prop : Outport
  wires:
  [rho] -> Propeller Function/5(density)
  MATLAB Function/2(alpha_prop) -> [alpha_prop]
  MATLAB Function/3(beta_prop) -> [beta_prop]
  MATLAB Function/1(TAS_prop) -> [TAS_prop]
  MATLAB Function/4(DCM_prop2b) -> [DCM_prop2b]
  tilt angle propeller/1 -> MATLAB Function/4(tilt_prop)
  [TAS_prop] -> Propeller Function/1(V)
  From CG/1 -> MATLAB Function/3(prop_pos)
  [alpha_prop] -> Propeller Function/3(alpha)
  rad/s propeller/1 -> speed limits/1
  States/1 -> Bus Selector/1
  Bus Selector/2 -> MATLAB Function/1(UVW)  "<Vb (m/s)>"
  Bus Selector/3 -> MATLAB Function/2(PQR)  "<w_b (rad/s)>"
  Bus Selector/1 -> [rho]  "<rho>"
  Mux/1 -> ForcesMoments_prop/1
  3x3 Cross Product/1 -> Sum/1
  Moments_prop to body axis/1 -> Sum/2  "Moments_prop"
  Forces_prop to body axis/1 -> 3x3 Cross Product/2, Mux/1  "Forces_prop"
  [DCM_prop2b] -> Forces_prop to body axis/1, Moments_prop to body axis/1
  From CG1/1 -> 3x3 Cross Product/1
  Bus Creator6/1 -> Moments_prop to body axis/2
  Bus Creator5/1 -> Forces_prop to body axis/2
  Sum/1 -> Mux/2
  [beta_prop] -> Propeller Function/4(beta)
  Constant/1 -> Propeller Function/7(Ap)
  Constant2/1 -> Propeller Function/6(Sn)
  Constant3/1 -> Propeller Function/8(pitch075)
  Constant4/1 -> Propeller Function/9(J_Table)
  Constant5/1 -> Propeller Function/10(CP_Table)
  Constant6/1 -> Propeller Function/11(CT_Table)
  Constant7/1 -> Propeller Function/13(sigma_e)
  "Coaxial "/1 -> Propeller Function/12(prop_type)
  Propeller Function/1(Forces) -> Demux/1
  Demux/1 -> Bus Creator5/1
  Demux/6 -> Bus Creator6/3
  Demux/2 -> Bus Creator5/2
  Demux/3 -> Bus Creator5/3
  Demux/5 -> Bus Creator6/2
  Propeller Function/2(Power) -> ?
  speed limits/1 -> Engine Lag/1
  Diameter/1 -> Propeller Function/14(D)
  rad/s to rps/1 -> Propeller Function/2(n)
  Coaxial propeller/1 -> Bus Creator6/1
  Engine Lag/1 -> rad/s to rps/1

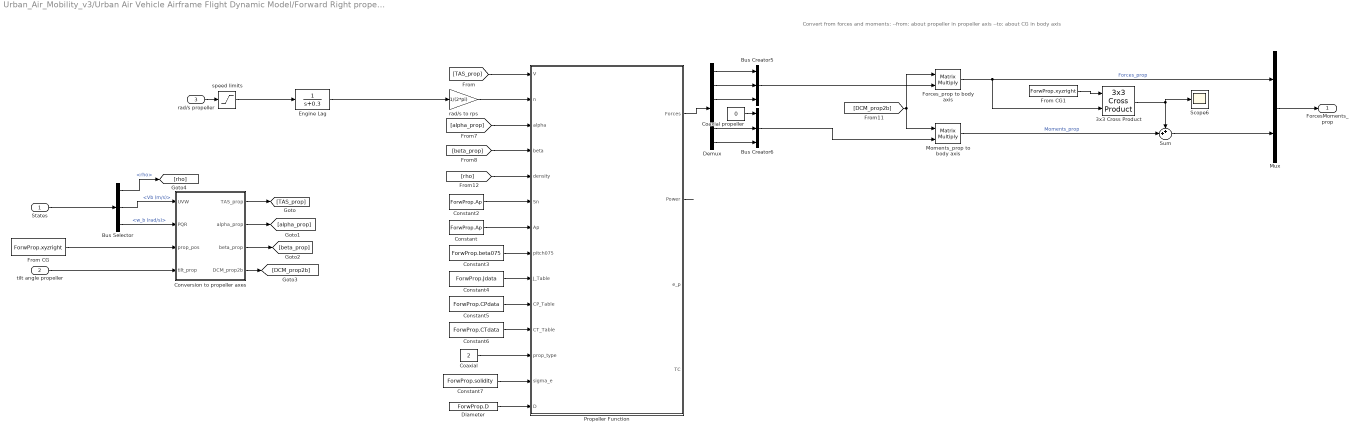
== system Urban_Air_Mobility_v3/Urban Air Vehicle Airframe Flight Dynamic Model/Forward Right propeller ==
  note: Convert from forces and moments: --from: about propeller in propeller axis --to: about CG in body axis
  States : Inport
  tilt angle propeller : Inport  Port=2
  rad/s propeller : Inport  Port=3
  3x3 Cross Product : sharedutil/3x3 Cross Product  aMode=aMode
      settings: SourceProductBaseCode=AE,PW,DR,MT,UV,VE
  Bus Creator5 : BusCreator  Inputs=3
  Bus Creator6 : BusCreator  Inputs=3
  Bus Selector : BusSelector  OutputSignals=rho,Vb (m/s),w_b (rad/s)
  "Coaxial " : Constant  Value=2
  Coaxial propeller : Constant  Value=0
  Constant : Constant  Value=ForwProp.Ap
  Constant2 : Constant  Value=ForwProp.Ap
  Constant3 : Constant  Value=ForwProp.beta075
  Constant4 : Constant  Value=ForwProp.Jdata
  Constant5 : Constant  Value=ForwProp.CPdata
  Constant6 : Constant  Value=ForwProp.CTdata
  Constant7 : Constant  Value=ForwProp.solidity
  Conversion to propeller axes : MATLAB Function  TreatAsAtomicUnit=on
  Demux : Demux  Outputs=6
  Diameter : Constant  Value=ForwProp.D
  Engine Lag : TransferFcn  Denominator=[1 0.3]  ContinuousStateAttributes='EngineLag'
  Forces_prop to body axis : Product  Multiplication=Matrix(*)
  From CG : Constant  Value=ForwProp.xyzright
  From CG1 : Constant  Value=ForwProp.xyzright
  Moments_prop to body axis : Product  Multiplication=Matrix(*)
  Mux : Mux  Inputs=2
  Propeller Function : MATLAB Function  TreatAsAtomicUnit=on
  Scope6 : Scope
  Sum : Sum  Inputs=++|
  rad/s to rps : Gain  Gain=1/(2*pi)
  speed limits : Saturate  UpperLimit=2000  LowerLimit=-1500
  ForcesMoments_prop : Outport
  wires:
  [rho] -> Propeller Function/5(density)
  Conversion to propeller axes/2(alpha_prop) -> [alpha_prop]
  Conversion to propeller axes/3(beta_prop) -> [beta_prop]
  Conversion to propeller axes/1(TAS_prop) -> [TAS_prop]
  Conversion to propeller axes/4(DCM_prop2b) -> [DCM_prop2b]
  tilt angle propeller/1 -> Conversion to propeller axes/4(tilt_prop)
  [TAS_prop] -> Propeller Function/1(V)
  speed limits/1 -> Engine Lag/1
  From CG/1 -> Conversion to propeller axes/3(prop_pos)
  [alpha_prop] -> Propeller Function/3(alpha)
  rad/s propeller/1 -> speed limits/1
  States/1 -> Bus Selector/1
  Bus Selector/2 -> Conversion to propeller axes/1(UVW)  "<Vb (m/s)>"
  Bus Selector/3 -> Conversion to propeller axes/2(PQR)  "<w_b (rad/s)>"
  Bus Selector/1 -> [rho]  "<rho>"
  Mux/1 -> ForcesMoments_prop/1
  3x3 Cross Product/1 -> Scope6/1, Sum/1
  Moments_prop to body axis/1 -> Sum/2  "Moments_prop"
  Forces_prop to body axis/1 -> 3x3 Cross Product/2, Mux/1  "Forces_prop"
  [DCM_prop2b] -> Forces_prop to body axis/1, Moments_prop to body axis/1
  From CG1/1 -> 3x3 Cross Product/1
  Bus Creator6/1 -> Moments_prop to body axis/2
  Bus Creator5/1 -> Forces_prop to body axis/2
  Sum/1 -> Mux/2
  [beta_prop] -> Propeller Function/4(beta)
  Constant/1 -> Propeller Function/7(Ap)
  Constant2/1 -> Propeller Function/6(Sn)
  Constant3/1 -> Propeller Function/8(pitch075)
  Constant4/1 -> Propeller Function/9(J_Table)
  Constant5/1 -> Propeller Function/10(CP_Table)
  Constant6/1 -> Propeller Function/11(CT_Table)
  Constant7/1 -> Propeller Function/13(sigma_e)
  "Coaxial "/1 -> Propeller Function/12(prop_type)
  Propeller Function/1(Forces) -> Demux/1
  Demux/1 -> Bus Creator5/1
  Demux/6 -> Bus Creator6/3
  Demux/3 -> Bus Creator5/3
  Demux/5 -> Bus Creator6/2
  Propeller Function/2(Power) -> ?
  Engine Lag/1 -> rad/s to rps/1
  Diameter/1 -> Propeller Function/14(D)
  rad/s to rps/1 -> Propeller Function/2(n)
  Coaxial propeller/1 -> Bus Creator6/1
  Demux/2 -> Bus Creator5/2

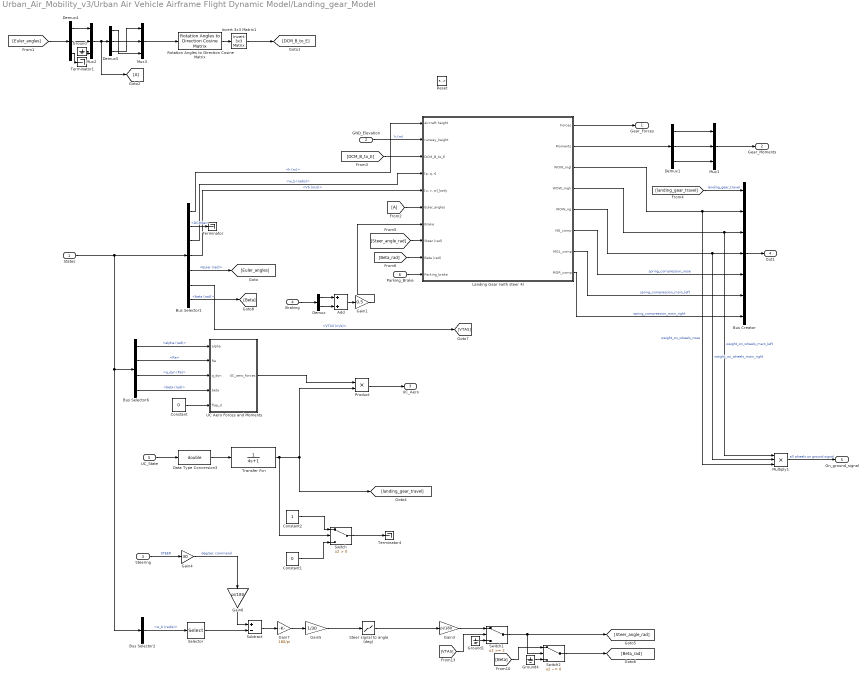
== system Urban_Air_Mobility_v3/Urban Air Vehicle Airframe Flight Dynamic Model/Landing_gear_Model ==
  States : Inport
  GND_Elevation : Inport  Port=2
  Steering : Inport  Port=3
  Braking : Inport  Port=4
  UC_State : Inport  Port=5
  Parking_Brake : Inport  Port=6
  Reset : ResetPort  DisableCoverage=on
  Add : Sum
  Bus Creator : BusCreator  Inputs=7
  Bus Selector1 : BusSelector  OutputSignals=h (m),DCMbe,w_b (rad/s),Vb (m/s),Euler (rad),VTAS (m/s),beta (rad)
  Bus Selector2 : BusSelector  OutputSignals=w_b (rad/s)
  Bus Selector6 : BusSelector  OutputSignals=alpha (rad),Re,q_dyn (Pa),beta (rad)
  Constant : Constant  Value=0
  Constant1 : Constant  Value=0
  Constant2 : Constant
  Data Type Conversion3 : DataTypeConversion  OutDataTypeStr=double
  Demux : Demux  Outputs=2
  Demux1 : Demux  Outputs=3
  Demux4 : Demux  Outputs=3
  Demux5 : Demux  Outputs=3
  Gain1 : Gain  Gain=0.5
  Gain3 : Gain  Gain=pi/180
  Gain4 : Gain  Gain=30
  Gain5 : Gain  Gain=1/30
  Gain6 : Gain  Gain=pi/180
  Gain7 : Gain  Gain=180/pi
  Ground : Ground
  Ground1 : Ground
  Ground4 : Ground
  Invert 3x3 Matrix1 : aerolibutil/Invert  3x3 Matrix
  Landing Gear (with steer 4) : Subsystem
  Multiply1 : Product  Inputs=3
  Mux1 : Mux  Inputs=3
  Mux2 : Mux  Inputs=3
  Mux3 : Mux  Inputs=3
  Product : Product
  Rotation Angles to Direction Cosine Matrix : sharedtransform/Rotation Angles to Direction Cosine Matrix  rotationOrder=ZYX  aMode=aMode
      settings: SourceProductBaseCode=AE,PW,DR,MT,UV,VE
  Selector : Selector  InputPortWidth=3  IndexOptions=Index vector (dialog)  Indices=3  OutputSizes=1
  Steer signal to angle (deg) : Lookup  InputValues=[-1 1]  Table=[-50 50]
  Subtract : Sum  Inputs=+-
  Switch : Switch  Criteria=u2 > Threshold
  Switch1 : Switch  Threshold=2
  Switch2 : Switch  Criteria=u2 ~= 0  Threshold=2
  Terminator : Terminator
  Terminator1 : Terminator
  Terminator4 : Terminator
  Transfer Fcn : TransferFcn  Denominator=[4 1]
  UC Aero Forces and Moments : Subsystem
  Gear_Forces : Outport  VectorParamsAs1DForOutWhenUnconnected=off
  Gear_Moments : Outport  Port=2  VectorParamsAs1DForOutWhenUnconnected=off
  UC_Aero : Outport  Port=3  VectorParamsAs1DForOutWhenUnconnected=off
  Out1 : Outport  Port=4  VectorParamsAs1DForOutWhenUnconnected=off
  On_ground_signal : Outport  Port=5  VectorParamsAs1DForOutWhenUnconnected=off
  wires:
  Bus Selector6/3 -> UC Aero Forces and Moments/3(q_dyn)  "<q_dyn (Pa)>"
  States/1 -> Bus Selector2/1, Bus Selector6/1, Bus Selector1/1
  Data Type Conversion3/1 -> Transfer Fcn/1
  Switch/1 -> Terminator4/1
  Constant/1 -> UC Aero Forces and Moments/5(flap_d)
  UC_State/1 -> Data Type Conversion3/1
  Constant1/1 -> Switch/3
  Transfer Fcn/1 -> Switch/2, Product/2, [landing_gear_travel]
  Constant2/1 -> Switch/1
  Bus Selector1/1 -> Landing Gear (with steer 4)/1(aircraft height)  "<h (m)>"
  GND_Elevation/1 -> Landing Gear (with steer 4)/2(runway_height)  "h (m)"
  Landing Gear (with steer 4)/2(Moments) -> Demux1/1
  Bus Selector1/4 -> Landing Gear (with steer 4)/5("[u, v, w]_body")  "<Vb (m/s)>"
  Demux/1 -> Add/1
  Demux/2 -> Add/2
  Add/1 -> Gain1/1
  Bus Selector1/6 -> [VTAS]  "<VTAS (m/s)>"
  Braking/1 -> Demux/1
  Gain1/1 -> Landing Gear (with steer 4)/7("Brake ")
  Demux1/2 -> Mux1/2
  Demux1/1 -> Mux1/1
  Mux1/1 -> Gear_Moments/1
  Steering/1 -> Gain4/1  "STEER"
  Landing Gear (with steer 4)/1("Forces ") -> Gear_Forces/1
  Bus Selector1/5 -> [Euler_angles]  "<Euler (rad)>"
  [Euler_angles] -> Demux4/1
  Demux4/2 -> Mux2/2
  Demux4/1 -> Mux2/1
  Ground/1 -> Mux2/3
  Mux2/1 -> [A], Demux5/1
  Demux5/3 -> Mux3/1
  Demux5/2 -> Mux3/2
  Demux5/1 -> Mux3/3
  Mux3/1 -> Rotation Angles to Direction Cosine Matrix/1
  Rotation Angles to Direction Cosine Matrix/1 -> Invert 3x3 Matrix1/1
  Invert 3x3 Matrix1/1 -> [DCM_B_to_E]
  [A] -> Landing Gear (with steer 4)/6(Euler_angles)
  [DCM_B_to_E] -> Landing Gear (with steer 4)/3(DCM_B_to_E)
  Bus Creator/1 -> Out1/1
  Landing Gear (with steer 4)/3(WOW_mgl) -> Multiply1/3, Bus Creator/2  "weight_on_wheels_nose"
  Landing Gear (with steer 4)/5("WOW_ng ") -> Multiply1/2, Bus Creator/4  "weight_on_wheels_main_right"
  Landing Gear (with steer 4)/6(NG_comp) -> Bus Creator/5  "spring_compression_nose"
  Landing Gear (with steer 4)/7(MGL_comp) -> Bus Creator/6  "spring_compression_main_left"
  Landing Gear (with steer 4)/8(MGR_comp) -> Bus Creator/7  "spring_compression_main_right"
  Landing Gear (with steer 4)/4(WOW_mglr) -> Multiply1/1, Bus Creator/3  "weight_on_wheels_main_left"
  [landing_gear_travel] -> Bus Creator/1  "landing_gear_travel"
  Demux1/3 -> Mux1/3
  Bus Selector1/3 -> Landing Gear (with steer 4)/4("[p, q, r]")  "<w_b (rad/s)>"
  Ground1/1 -> Switch1/3
  Gain3/1 -> Switch1/1
  [VTAS] -> Switch1/2
  Switch1/1 -> [Steer_angle_rad], Switch2/2
  Switch2/1 -> [Beta_rad]
  Ground4/1 -> Switch2/3
  [Beta] -> Switch2/1
  Bus Selector1/7 -> [Beta]  "<beta (rad)>"
  Steer signal to angle (deg)/1 -> Gain3/1
  [Steer_angle_rad] -> Landing Gear (with steer 4)/8("Steer (rad) ")
  [Beta_rad] -> Landing Gear (with steer 4)/9("Beta (rad) ")
  Parking_Brake/1 -> Landing Gear (with steer 4)/10(Parking_brake)
  Bus Selector2/1 -> Selector/1  "<w_b (rad/s)>"
  Selector/1 -> Subtract/2
  Gain4/1 -> Gain6/1  "deg/sec command"
  Subtract/1 -> Gain7/1
  Gain5/1 -> Steer signal to angle (deg)/1
  Gain6/1 -> Subtract/1
  Gain7/1 -> Gain5/1
  Multiply1/1 -> On_ground_signal/1  "all wheels on ground signal"
  Demux4/3 -> Terminator1/1
  Bus Selector1/2 -> Terminator/1  "<DCMbe>"
  Bus Selector6/2 -> UC Aero Forces and Moments/2(Re)  "<Re>"
  Bus Selector6/1 -> UC Aero Forces and Moments/1(alpha)  "<alpha (rad)>"
  UC Aero Forces and Moments/1(UC_aero_forces) -> Product/1
  Bus Selector6/4 -> UC Aero Forces and Moments/4(beta)  "<beta (rad)>"
  Product/1 -> UC_Aero/1
